simulink model "quad_nolinear"  (R2017b)
settings: Solver=VariableStepAuto  StartTime=0.0  StopTime=280  RelTol=1e-3
values from neighbouring files (symbols this model uses):
  A11 = Ab(1:6,1:6)    [quadrirrotor_ws.m]
  A12 = Ab(1:6,7:12)    [quadrirrotor_ws.m]
  A21 = Ab(7:12,1:6)    [quadrirrotor_ws.m]
  A22 = Ab(7:12,7:12)    [quadrirrotor_ws.m]
  Am = [zeros(6) eye(6); A_l zeros(6)]    [quadrirrotor_ws.m]
  B1 = Bb(1:6,:)    [quadrirrotor_ws.m]
  B2 = Bb(7:12,:)    [quadrirrotor_ws.m]
  Bm = [zeros(8,4); 1/m 0 0 0;0 1/Ixx 0 0;0 0 1/Iyy 0;0 0 0 1/Izz]    [quadrirrotor_ws.m]
  Cm = [eye(6) zeros(6)]    [quadrirrotor_ws.m]
  Dm = zeros(6,4)    [quadrirrotor_ws.m]
  g = 9.81    [quadrirrotor_ws.m]
  Ixx = 0.0363    [quadrirrotor_ws.m]
  Iyy = 0.0363    [quadrirrotor_ws.m]
  Izz = 0.0615    [quadrirrotor_ws.m]
  K = inv(R)*B'*P    [quadrirrotor_ws.m]
  Km = [zeros(6,12) ... (first row only)    [quadrirrotor_ws.m]
  Lb = inv(T)*Lc    [quadrirrotor_ws.m]
  m = 2.24    [quadrirrotor_ws.m]
  Y1 = Y(:,1:6)    [quadrirrotor_ws.m]
  Y2 = Y(:,7:12)    [quadrirrotor_ws.m]
libraries: simulink x4
settings Model: Creator=Italo  LastModifiedBy=Italo
settings OptimizationCC: LifeSpan=inf
settings DebuggingCC: SFExecutionAtInitializationDiag=none
settings CodeAppCC: StateflowObjectComments=on

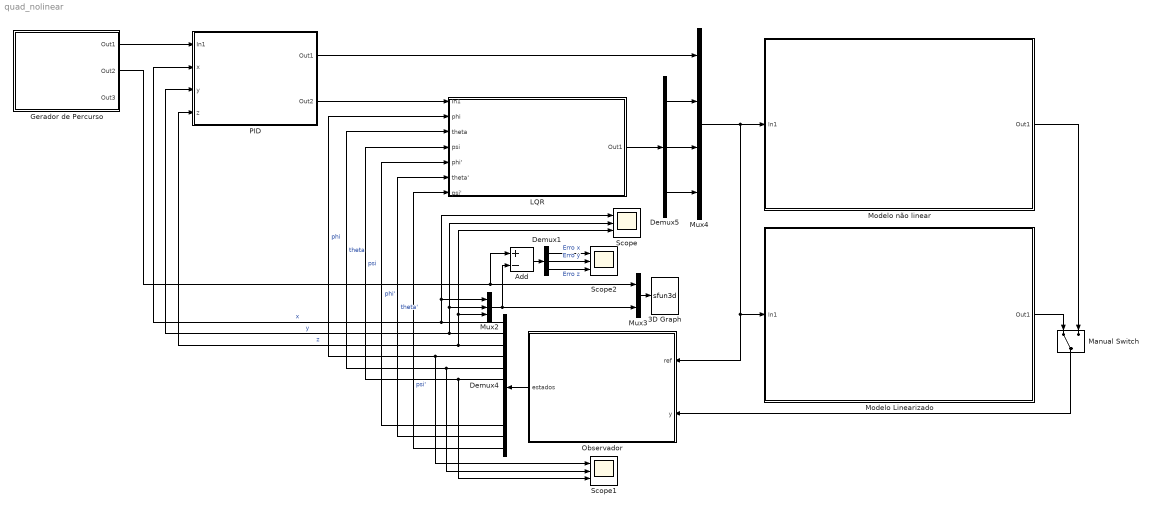
== system quad_nolinear ==
  3D Graph : S-Function  LoadFcn=if exist('sfun3d','file'), sfun3d([],[],[],'LoadBlock'); end  FunctionName=sfun3d  Parameters=ax,T,np,cp,gd,ls,mk,mx,hd,tb  SFunctionDeploymentMode=off  EnableBusSupport=off  mask(3D Graph){np=2, ax=[-5 5 -5 5 0 1500], mx=1e4, T=0.1, cp=[3 2 1], gd=on, hd=off, tb=off, ls=--, mk=none}
      mask prompts: np "Number of moving points (lines)"; ax "Range: [xmin xmax  ymin ymax zmin zmax]"; mx "Max number of points in each line"; T "Sampling Time"; cp "Camera position (use [0 0 1] for 2D XY view)"; gd "Grid (on|off)"; hd "HeadMarkers (on|off)"; tb "Toolbar (on|off)"; ls "LineStyle"; mk "LineMarker"
      mask help:
      | This block plots the position of several points in the XYZ space. The input contains the coordinates of all the points (x1,y1,z1,x2,y2,z2,...).
      | The number of moving points (lines), the XYZ ranges, sampling time, camera position, and grid (among other things) can be set as mask parameters.
      settings: CopyFcn=if exist('sfun3d','file'), sfun3d([],[],[],'CopyBlock'); end  DeleteFcn=if exist('sfun3d','file'), sfun3d([],[],[],'DeleteBlock'); end  NameChangeFcn=if exist('sfun3d','file'), sfun3d([],[],[],'NameChange'); end
      mask Help:
      | This block plots the position of several points in the XYZ space. The input contains the coordinates of all the points (x1,y1,z1,x2,y2,z2,...).
      | The number of moving points (lines), the XYZ ranges, sampling time, camera position, and grid (among other things) can be set as mask parameters.
      mask TypeOptions ls: - | -- | : | -. | none
      mask TypeOptions mk: none | . | + | o | * | x | square | diamond | v | ^ | > | < | pentagram | hexagram
      mask Display: plot([.05 .95 .95 .05 .05],[.45 .45 .95 .95 .45], 0.5+cos(0:0.1:2*pi)*0.3,0.7+sin(0:0.1:2*pi)*0.2)
  Add : Sum  Inputs=+-
  Demux1 : Demux  Outputs=3
  Demux4 : Demux  Outputs=12
  Demux5 : Demux  Outputs=3
  Gerador de Percurso : Subsystem
      mask Display: image('gerador.jpg');
  LQR : Subsystem
      mask Display: image('lqr.png');
  Manual Switch : ManualSwitch
  Modelo Linearizado : Subsystem
      mask Display: image('quadrotor.jpg');
  Modelo não linear : Subsystem
      mask Display: image('quadrotor.jpg');
  Mux2 : Mux  Inputs=3
  Mux3 : Mux  Inputs=2
  Mux4 : Mux
  Observador : Subsystem
      mask Display: image('observador.jpg');
  PID : Subsystem
      mask Display: image('pid.jpg');
  Scope : Scope  NumInputPorts=3
  Scope1 : Scope  NumInputPorts=3
  Scope2 : Scope  NumInputPorts=3
  wires:
  Demux5/3 -> Mux4/4
  Demux4/3 -> Mux2/3, Scope/3, PID/4(z)  "z"
  Demux4/6 -> Scope1/3, LQR/4(psi)  "psi"
  Demux4/2 -> Mux2/2, Scope/2, PID/3(y)  "y"
  Demux4/1 -> Mux2/1, Scope/1, PID/2(x)  "x"
  Demux5/1 -> Mux4/2
  Demux4/5 -> Scope1/2, LQR/3(theta)  "theta"
  Demux4/4 -> Scope1/1, LQR/2(phi)  "phi"
  Mux4/1 -> Observador/1(ref), Modelo Linearizado/1(In1), Modelo não linear/1(In1)
  Observador/1("estados ") -> Demux4/1
  Demux5/2 -> Mux4/3
  Manual Switch/1 -> Observador/2(y)
  Modelo Linearizado/1(Out1) -> Manual Switch/1
  Mux3/1 -> 3D Graph/1
  Mux2/1 -> Mux3/2, Add/2
  Gerador de Percurso/2(Out2) -> Add/1, Mux3/1
  Gerador de Percurso/1(Out1) -> PID/1(In1)
  PID/1(Out1) -> Mux4/1
  PID/2(Out2) -> LQR/1(In1)
  Demux4/10 -> LQR/5(phi')  "phi'"
  Demux4/11 -> LQR/6(theta')  "theta'"
  Demux4/12 -> LQR/7(psi')  "psi'"
  LQR/1(Out1) -> Demux5/1
  Add/1 -> Demux1/1
  Demux1/1 -> Scope2/1  "Erro x"
  Demux1/2 -> Scope2/2  "Erro y"
  Demux1/3 -> Scope2/3  "Erro z"
  Modelo não linear/1(Out1) -> Manual Switch/2

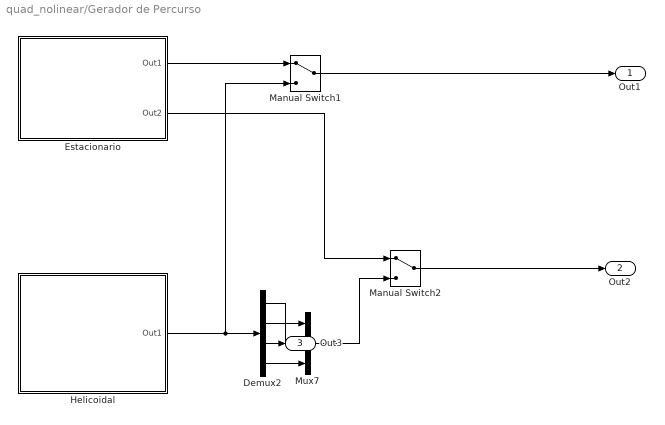
== system quad_nolinear/Gerador de Percurso ==
  Demux2 : Demux
  Estacionario : Subsystem
  Helicoidal : Subsystem
  Manual Switch1 : ManualSwitch
  Manual Switch2 : ManualSwitch
  Mux7 : Mux  Inputs=3
  Out1 : Outport
  Out2 : Outport  Port=2
  Out3 : Outport  Port=3
  wires:
  Manual Switch1/1 -> Out1/1
  Helicoidal/1(Out1) -> Manual Switch1/2, Demux2/1
  Manual Switch2/1 -> Out2/1
  Demux2/2 -> Mux7/1
  Demux2/3 -> Out3/1
  Demux2/4 -> Mux7/3
  Mux7/1 -> Manual Switch2/2
  Estacionario/1(Out1) -> Manual Switch1/1
  Estacionario/2(Out2) -> Manual Switch2/1
  Demux2/1 -> Mux7/2

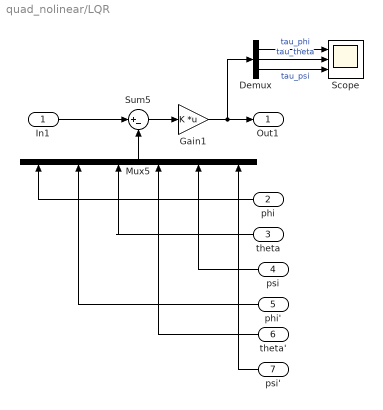
== system quad_nolinear/LQR ==
  In1 : Inport
  phi : Inport  Port=2
  theta : Inport  Port=3
  psi : Inport  Port=4
  phi' : Inport  Port=5
  theta' : Inport  Port=6
  psi' : Inport  Port=7
  Demux : Demux  Outputs=3
  Gain1 : Gain  Gain=K  Multiplication=Matrix(K*u) (u vector)
  Mux5 : Mux  Inputs=6
  Scope : Scope  NumInputPorts=3
  Sum5 : Sum  Inputs=|+-
  Out1 : Outport
  wires:
  theta/1 -> Mux5/3
  phi/1 -> Mux5/1
  psi/1 -> Mux5/5
  theta'/1 -> Mux5/4
  Sum5/1 -> Gain1/1
  psi'/1 -> Mux5/6
  phi'/1 -> Mux5/2
  Gain1/1 -> Demux/1, Out1/1
  Mux5/1 -> Sum5/2
  In1/1 -> Sum5/1
  Demux/1 -> Scope/1  "tau_phi"
  Demux/2 -> Scope/2  "tau_theta"
  Demux/3 -> Scope/3  "tau_psi"

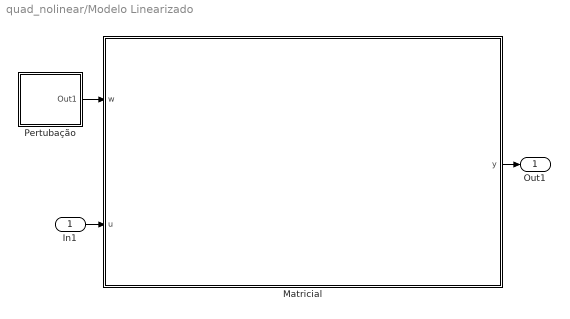
== system quad_nolinear/Modelo Linearizado ==
  In1 : Inport
  Matricial : Subsystem
  Pertubação : Subsystem
  Out1 : Outport
  wires:
  Pertubação/1(Out1) -> Matricial/1(w)
  In1/1 -> Matricial/2(u)
  Matricial/1(y) -> Out1/1

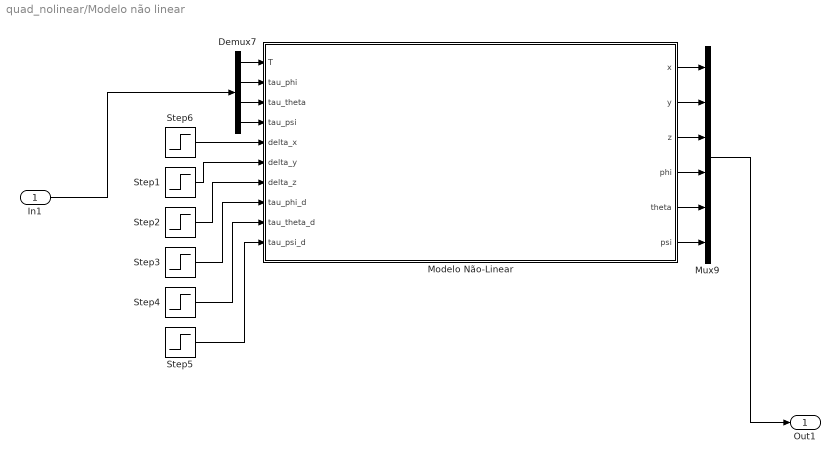
== system quad_nolinear/Modelo não linear ==
  In1 : Inport
  Demux7 : Demux
  Modelo Não-Linear : Subsystem
  Mux9 : Mux  Inputs=6
  Step1 : Step  Time=250  After=0.5  SampleTime=0
  Step2 : Step  Time=300  After=0.5  SampleTime=0
  Step3 : Step  Time=350  After=0.5  SampleTime=0
  Step4 : Step  Time=400  After=0.5  SampleTime=0
  Step5 : Step  Time=450  After=0.5  SampleTime=0
  Step6 : Step  Time=200  After=0.5  SampleTime=0
  Out1 : Outport
  wires:
  Modelo Não-Linear/1(x) -> Mux9/1
  In1/1 -> Demux7/1
  Step6/1 -> Modelo Não-Linear/5(delta_x)
  Step1/1 -> Modelo Não-Linear/6(delta_y)
  Step2/1 -> Modelo Não-Linear/7(delta_z)
  Step4/1 -> Modelo Não-Linear/9(tau_theta_d)
  Step5/1 -> Modelo Não-Linear/10(tau_psi_d)
  Step3/1 -> Modelo Não-Linear/8(tau_phi_d)
  Modelo Não-Linear/6(psi) -> Mux9/6
  Modelo Não-Linear/4(phi) -> Mux9/4
  Mux9/1 -> Out1/1
  Modelo Não-Linear/2(y) -> Mux9/2
  Modelo Não-Linear/3(z) -> Mux9/3
  Modelo Não-Linear/5(theta) -> Mux9/5
  Demux7/4 -> Modelo Não-Linear/4(tau_psi)
  Demux7/3 -> Modelo Não-Linear/3(tau_theta)
  Demux7/1 -> Modelo Não-Linear/1(T)
  Demux7/2 -> Modelo Não-Linear/2(tau_phi)

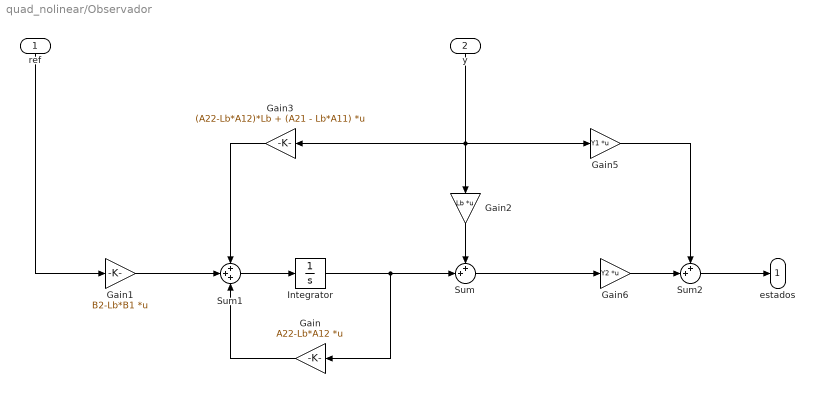
== system quad_nolinear/Observador ==
  ref : Inport
  y : Inport  Port=2
  Gain : Gain  Gain=A22-Lb*A12  Multiplication=Matrix(K*u) (u vector)
  Gain1 : Gain  Gain=B2-Lb*B1  Multiplication=Matrix(K*u) (u vector)
  Gain2 : Gain  Gain=Lb  Multiplication=Matrix(K*u) (u vector)
  Gain3 : Gain  Gain=(A22-Lb*A12)*Lb + (A21 - Lb*A11)  Multiplication=Matrix(K*u) (u vector)
  Gain5 : Gain  Gain=Y1  Multiplication=Matrix(K*u) (u vector)
  Gain6 : Gain  Gain=Y2  Multiplication=Matrix(K*u) (u vector)
  Integrator : Integrator
  Sum : Sum  Inputs=++|
  Sum1 : Sum  Inputs=+++
  Sum2 : Sum  Inputs=++|
  "estados " : Outport
  wires:
  Sum1/1 -> Integrator/1
  Integrator/1 -> Sum/2, Gain/1
  Gain/1 -> Sum1/3
  ref/1 -> Gain1/1
  Gain1/1 -> Sum1/2
  Gain3/1 -> Sum1/1
  y/1 -> Gain5/1, Gain3/1, Gain2/1
  Gain2/1 -> Sum/1
  Sum/1 -> Gain6/1
  Gain6/1 -> Sum2/2
  Sum2/1 -> "estados "/1
  Gain5/1 -> Sum2/1

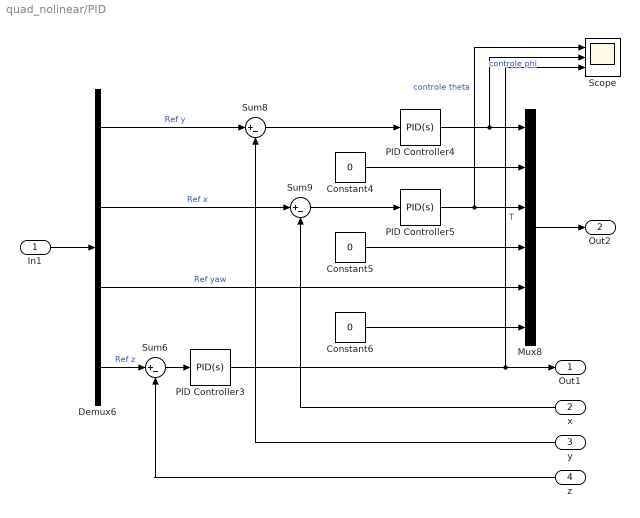
== system quad_nolinear/PID ==
  In1 : Inport
  x : Inport  Port=2
  y : Inport  Port=3
  z : Inport  Port=4
  Constant4 : Constant  Value=0
  Constant5 : Constant  Value=0
  Constant6 : Constant  Value=0
  Demux6 : Demux
  Mux8 : Mux  Inputs=6
  PID Controller3 : simulink/Continuous/PID Controller  Controller=PID  TimeDomain=Continuous-time  SampleTime=-1  IntegratorMethod=Forward Euler  FilterMethod=Forward Euler  Form=Ideal  UseFilter=on  ControllerParametersSource=internal  P=0.4  I=0.04  D=5.56  N=5.46  InitialConditionSource=internal  InitialConditionForIntegrator=0  InitialConditionForFilter=0  ExternalReset=none  LimitOutput=off  UpperSaturationLimit=inf  LowerSaturationLimit=-inf  LinearizeAsGain=on  AntiWindupMode=none  Kb=1  TrackingMode=off  Kt=1  PParamMin=[]  PParamMax=[]  IParamMin=[]  IParamMax=[]  DParamMin=[]  DParamMax=[]  NParamMin=[]  NParamMax=[]  KbParamMin=[]  KbParamMax=[]  KtParamMin=[]  KtParamMax=[]  POutMin=[]  POutMax=[]  IOutMin=[]  IOutMax=[]  DOutMin=[]  DOutMax=[]  NOutMin=[]  NOutMax=[]  KbOutMin=[]  KbOutMax=[]  KtOutMin=[]  KtOutMax=[]  IntegratorOutMin=[]  IntegratorOutMax=[]  FilterOutMin=[]  FilterOutMax=[]  SumOutMin=[]  SumOutMax=[]  SumI1OutMin=[]  SumI1OutMax=[]  SumI2OutMin=[]  SumI2OutMax=[]  SumI3OutMin=[]  SumI3OutMax=[]  SumDOutMin=[]  SumDOutMax=[]  SaturationOutMin=[]  SaturationOutMax=[]  IntegratorContinuousStateAttributes=''  IntegratorStateMustResolveToSignalObject=off  IntegratorRTWStateStorageClass=Auto  FilterContinuousStateAttributes=''  FilterStateMustResolveToSignalObject=off  FilterRTWStateStorageClass=Auto  DifferentiatorICPrevScaledInput=0  DifferentiatorOutMin=[]  DifferentiatorOutMax=[]  InitialConditionSetting=State (most efficient)  FilterDiffOutCoefMin=[]  FilterDiffOutCoefMax=[]  SumDenOutMin=[]  SumDenOutMax=[]  SumNumOutMin=[]  SumNumOutMax=[]  ReciprocalOutMin=[]  ReciprocalOutMax=[]  DivideOutMin=[]  DivideOutMax=[]  TunerSelectOption=Transfer Function Based (PID Tuner App)
  PID Controller4 : simulink/Continuous/PID Controller  Controller=PID  TimeDomain=Continuous-time  SampleTime=-1  IntegratorMethod=Forward Euler  FilterMethod=Forward Euler  Form=Ideal  UseFilter=on  ControllerParametersSource=internal  P=-0.01  I=0.01  D=30  N=140  InitialConditionSource=internal  InitialConditionForIntegrator=0  InitialConditionForFilter=0  ExternalReset=none  LimitOutput=off  UpperSaturationLimit=inf  LowerSaturationLimit=-inf  LinearizeAsGain=on  AntiWindupMode=none  Kb=1  TrackingMode=off  Kt=1  PParamMin=[]  PParamMax=[]  IParamMin=[]  IParamMax=[]  DParamMin=[]  DParamMax=[]  NParamMin=[]  NParamMax=[]  KbParamMin=[]  KbParamMax=[]  KtParamMin=[]  KtParamMax=[]  POutMin=[]  POutMax=[]  IOutMin=[]  IOutMax=[]  DOutMin=[]  DOutMax=[]  NOutMin=[]  NOutMax=[]  KbOutMin=[]  KbOutMax=[]  KtOutMin=[]  KtOutMax=[]  IntegratorOutMin=[]  IntegratorOutMax=[]  FilterOutMin=[]  FilterOutMax=[]  SumOutMin=[]  SumOutMax=[]  SumI1OutMin=[]  SumI1OutMax=[]  SumI2OutMin=[]  SumI2OutMax=[]  SumI3OutMin=[]  SumI3OutMax=[]  SumDOutMin=[]  SumDOutMax=[]  SaturationOutMin=[]  SaturationOutMax=[]  IntegratorContinuousStateAttributes=''  IntegratorStateMustResolveToSignalObject=off  IntegratorRTWStateStorageClass=Auto  FilterContinuousStateAttributes=''  FilterStateMustResolveToSignalObject=off  FilterRTWStateStorageClass=Auto  DifferentiatorICPrevScaledInput=0  DifferentiatorOutMin=[]  DifferentiatorOutMax=[]  InitialConditionSetting=State (most efficient)  FilterDiffOutCoefMin=[]  FilterDiffOutCoefMax=[]  SumDenOutMin=[]  SumDenOutMax=[]  SumNumOutMin=[]  SumNumOutMax=[]  ReciprocalOutMin=[]  ReciprocalOutMax=[]  DivideOutMin=[]  DivideOutMax=[]  TunerSelectOption=Transfer Function Based (PID Tuner App)
  PID Controller5 : simulink/Continuous/PID Controller  Controller=PID  TimeDomain=Continuous-time  SampleTime=-1  IntegratorMethod=Forward Euler  FilterMethod=Forward Euler  Form=Ideal  UseFilter=on  ControllerParametersSource=internal  P=0.001  I=0.003  D=60  N=58  InitialConditionSource=internal  InitialConditionForIntegrator=0  InitialConditionForFilter=0  ExternalReset=none  LimitOutput=off  UpperSaturationLimit=inf  LowerSaturationLimit=-inf  LinearizeAsGain=on  AntiWindupMode=none  Kb=1  TrackingMode=off  Kt=1  PParamMin=[]  PParamMax=[]  IParamMin=[]  IParamMax=[]  DParamMin=[]  DParamMax=[]  NParamMin=[]  NParamMax=[]  KbParamMin=[]  KbParamMax=[]  KtParamMin=[]  KtParamMax=[]  POutMin=[]  POutMax=[]  IOutMin=[]  IOutMax=[]  DOutMin=[]  DOutMax=[]  NOutMin=[]  NOutMax=[]  KbOutMin=[]  KbOutMax=[]  KtOutMin=[]  KtOutMax=[]  IntegratorOutMin=[]  IntegratorOutMax=[]  FilterOutMin=[]  FilterOutMax=[]  SumOutMin=[]  SumOutMax=[]  SumI1OutMin=[]  SumI1OutMax=[]  SumI2OutMin=[]  SumI2OutMax=[]  SumI3OutMin=[]  SumI3OutMax=[]  SumDOutMin=[]  SumDOutMax=[]  SaturationOutMin=[]  SaturationOutMax=[]  IntegratorContinuousStateAttributes=''  IntegratorStateMustResolveToSignalObject=off  IntegratorRTWStateStorageClass=Auto  FilterContinuousStateAttributes=''  FilterStateMustResolveToSignalObject=off  FilterRTWStateStorageClass=Auto  DifferentiatorICPrevScaledInput=0  DifferentiatorOutMin=[]  DifferentiatorOutMax=[]  InitialConditionSetting=State (most efficient)  FilterDiffOutCoefMin=[]  FilterDiffOutCoefMax=[]  SumDenOutMin=[]  SumDenOutMax=[]  SumNumOutMin=[]  SumNumOutMax=[]  ReciprocalOutMin=[]  ReciprocalOutMax=[]  DivideOutMin=[]  DivideOutMax=[]  TunerSelectOption=Transfer Function Based (PID Tuner App)
  Scope : Scope  NumInputPorts=3
  Sum6 : Sum  Inputs=|+-
  Sum8 : Sum  Inputs=|+-
  Sum9 : Sum  Inputs=|+-
  Out1 : Outport
  Out2 : Outport  Port=2
  wires:
  Demux6/2 -> Sum9/1  "Ref x"
  Demux6/4 -> Sum6/1  "Ref z"
  Mux8/1 -> Out2/1
  Sum9/1 -> PID Controller5/1
  Constant4/1 -> Mux8/2
  Demux6/1 -> Sum8/1  "Ref y"
  PID Controller3/1 -> Scope/3, Out1/1  "T"
  Sum6/1 -> PID Controller3/1
  Constant6/1 -> Mux8/6
  Constant5/1 -> Mux8/4
  Demux6/3 -> Mux8/5  "Ref yaw"
  Sum8/1 -> PID Controller4/1
  In1/1 -> Demux6/1
  PID Controller4/1 -> Scope/2, Mux8/1  "controle phi"
  y/1 -> Sum8/2
  x/1 -> Sum9/2
  z/1 -> Sum6/2
  PID Controller5/1 -> Scope/1, Mux8/3  "controle theta"

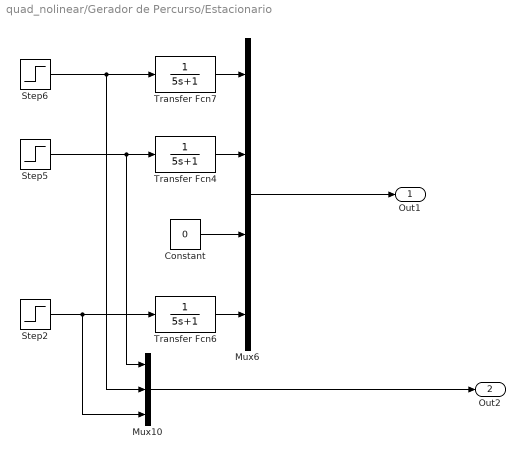
== system quad_nolinear/Gerador de Percurso/Estacionario ==
  Constant : Constant  Value=0
  Mux10 : Mux  Inputs=3
  Mux6 : Mux
  Step2 : Step  After=10  SampleTime=0
  Step5 : Step  After=2  SampleTime=0
  Step6 : Step  After=2  SampleTime=0
  Transfer Fcn4 : TransferFcn  Denominator=[5 1]
  Transfer Fcn6 : TransferFcn  Denominator=[5 1]
  Transfer Fcn7 : TransferFcn  Denominator=[5 1]
  Out1 : Outport
  Out2 : Outport  Port=2
  wires:
  Mux10/1 -> Out2/1
  Step2/1 -> Mux10/3, Transfer Fcn6/1
  Constant/1 -> Mux6/3
  Transfer Fcn7/1 -> Mux6/1
  Transfer Fcn4/1 -> Mux6/2
  Step6/1 -> Mux10/2, Transfer Fcn7/1
  Transfer Fcn6/1 -> Mux6/4
  Step5/1 -> Mux10/1, Transfer Fcn4/1
  Mux6/1 -> Out1/1

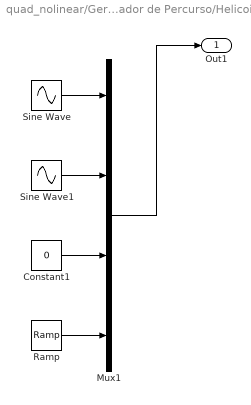
== system quad_nolinear/Gerador de Percurso/Helicoidal ==
  Constant1 : Constant  Value=0
  Mux1 : Mux
  Ramp : simulink/Sources/Ramp  slope=3  start=0  X0=1
  Sine Wave : Sin  Amplitude=3  Frequency=0.1  SampleTime=0
  Sine Wave1 : Sin  Amplitude=3  Frequency=0.1  Phase=pi/2  SampleTime=0
  Out1 : Outport
  wires:
  Sine Wave1/1 -> Mux1/2
  Sine Wave/1 -> Mux1/1
  Ramp/1 -> Mux1/4
  Mux1/1 -> Out1/1
  Constant1/1 -> Mux1/3

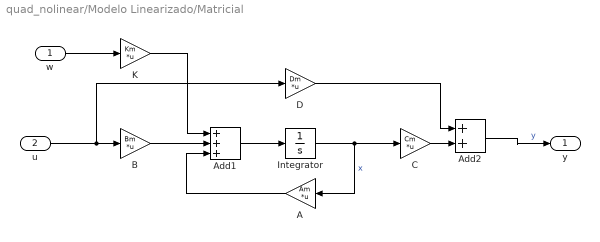
== system quad_nolinear/Modelo Linearizado/Matricial ==
  w : Inport
  u : Inport  Port=2
  A : Gain  Gain=Am  Multiplication=Matrix(K*u) (u vector)
  Add1 : Sum  Inputs=+++
  Add2 : Sum
  B : Gain  Gain=Bm  Multiplication=Matrix(K*u) (u vector)
  C : Gain  Gain=Cm  Multiplication=Matrix(K*u) (u vector)
  D : Gain  Gain=Dm  Multiplication=Matrix(K*u) (u vector)
  Integrator : Integrator
  K : Gain  Gain=Km  Multiplication=Matrix(K*u) (u vector)
  y : Outport
  wires:
  u/1 -> D/1, B/1
  Add2/1 -> y/1  "y"
  B/1 -> Add1/2
  Integrator/1 -> A/1, C/1  "x"
  A/1 -> Add1/3
  K/1 -> Add1/1
  D/1 -> Add2/1
  w/1 -> K/1
  Add1/1 -> Integrator/1
  C/1 -> Add2/2

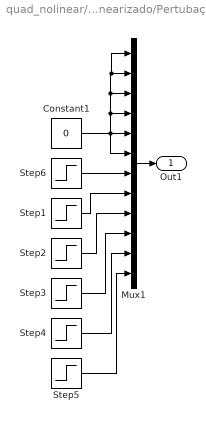
== system quad_nolinear/Modelo Linearizado/Pertubação ==
  Constant1 : Constant  Value=0
  Mux1 : Mux  Inputs=12
  Step1 : Step  Time=250  After=0.01  SampleTime=0
  Step2 : Step  Time=300  After=0.01  SampleTime=0
  Step3 : Step  Time=350  After=0.01  SampleTime=0
  Step4 : Step  Time=400  After=0.01  SampleTime=0
  Step5 : Step  Time=450  After=0.01  SampleTime=0
  Step6 : Step  Time=200  After=0.01  SampleTime=0
  Out1 : Outport
  wires:
  Step2/1 -> Mux1/9
  Step5/1 -> Mux1/12
  Mux1/1 -> Out1/1
  Constant1/1 -> Mux1/6, Mux1/1, Mux1/2, Mux1/3, Mux1/4, Mux1/5
  Step3/1 -> Mux1/10
  Step6/1 -> Mux1/7
  Step4/1 -> Mux1/11
  Step1/1 -> Mux1/8

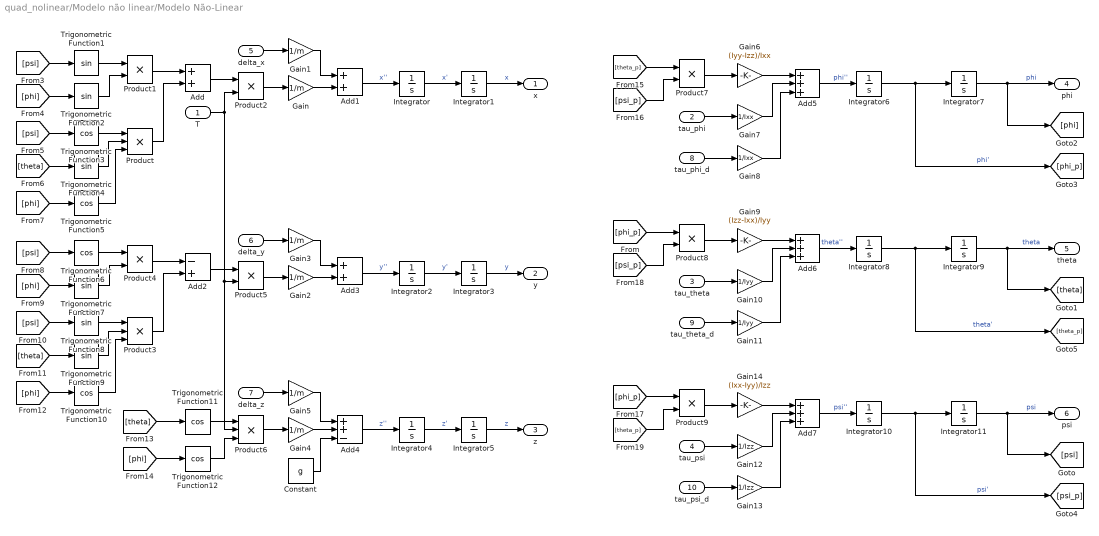
== system quad_nolinear/Modelo não linear/Modelo Não-Linear ==
  T : Inport
  tau_phi : Inport  Port=2
  tau_theta : Inport  Port=3
  tau_psi : Inport  Port=4
  delta_x : Inport  Port=5
  delta_y : Inport  Port=6
  delta_z : Inport  Port=7
  tau_phi_d : Inport  Port=8
  tau_theta_d : Inport  Port=9
  tau_psi_d : Inport  Port=10
  Add : Sum
  Add1 : Sum
  Add2 : Sum  Inputs=-+
  Add3 : Sum
  Add4 : Sum  Inputs=++-
  Add5 : Sum  Inputs=+++
  Add6 : Sum  Inputs=+++
  Add7 : Sum  Inputs=+++
  Constant : Constant  Value=g
  Gain{,1..5} (6 alike) : Gain  Gain=1/m
  Gain10 : Gain  Gain=1/Iyy
  Gain11 : Gain  Gain=1/Iyy
  Gain12 : Gain  Gain=1/Izz
  Gain13 : Gain  Gain=1/Izz
  Gain14 : Gain  Gain=(Ixx-Iyy)/Izz
  Gain6 : Gain  Gain=(Iyy-Izz)/Ixx
  Gain7 : Gain  Gain=1/Ixx
  Gain8 : Gain  Gain=1/Ixx
  Gain9 : Gain  Gain=(Izz-Ixx)/Iyy
  Integrator{,1..11} (12 alike) : Integrator
  Product : Product  Inputs=3
  Product{1..2,4..5,7..9} (7 alike) : Product
  Product3 : Product  Inputs=3
  Product6 : Product  Inputs=3
  Trigonometric Function{1..2,4,7..9} (6 alike) : Trigonometry
  Trigonometric Function{3,5..6,10..12} (6 alike) : Trigonometry  Operator=cos
  x : Outport
  y : Outport  Port=2
  z : Outport  Port=3
  phi : Outport  Port=4
  theta : Outport  Port=5
  psi : Outport  Port=6
  wires:
  Integrator/1 -> Integrator1/1  "x'"
  Integrator1/1 -> x/1  "x"
  Trigonometric Function1/1 -> Product1/1
  Trigonometric Function2/1 -> Product1/2
  [psi] -> Trigonometric Function1/1
  [phi] -> Trigonometric Function2/1
  Trigonometric Function3/1 -> Product/1
  [psi] -> Trigonometric Function3/1
  Trigonometric Function4/1 -> Product/2
  [theta] -> Trigonometric Function4/1
  Trigonometric Function5/1 -> Product/3
  [phi] -> Trigonometric Function5/1
  Product1/1 -> Add/1
  Product/1 -> Add/2
  Add/1 -> Product2/1
  Product2/1 -> Gain/1
  Gain/1 -> Add1/2
  Gain1/1 -> Add1/1
  Add1/1 -> Integrator/1  "x''"
  Integrator2/1 -> Integrator3/1  "y'"
  [psi] -> Trigonometric Function8/1
  Trigonometric Function9/1 -> Product3/2
  Product4/1 -> Add2/1
  [theta] -> Trigonometric Function9/1
  Add3/1 -> Integrator2/1  "y''"
  Trigonometric Function6/1 -> Product4/1
  Trigonometric Function10/1 -> Product3/3
  [psi] -> Trigonometric Function6/1
  Trigonometric Function7/1 -> Product4/2
  Gain2/1 -> Add3/2
  Product5/1 -> Gain2/1
  Integrator3/1 -> y/1  "y"
  [phi] -> Trigonometric Function10/1
  Product3/1 -> Add2/2
  Gain3/1 -> Add3/1
  Add2/1 -> Product5/1
  [phi] -> Trigonometric Function7/1
  Trigonometric Function8/1 -> Product3/1
  Product6/1 -> Gain4/1
  Add4/1 -> Integrator4/1  "z''"
  Gain4/1 -> Add4/2
  T/1 -> Product6/2, Product5/2, Product2/2
  Gain5/1 -> Add4/1
  Integrator4/1 -> Integrator5/1  "z'"
  Trigonometric Function11/1 -> Product6/1
  Integrator5/1 -> z/1  "z"
  Constant/1 -> Add4/3
  Trigonometric Function12/1 -> Product6/3
  [theta] -> Trigonometric Function11/1
  [phi] -> Trigonometric Function12/1
  Add5/1 -> Integrator6/1  "phi''"
  Integrator7/1 -> [phi], phi/1  "phi"
  Integrator6/1 -> Integrator7/1, [phi_p]  "phi'"
  Product7/1 -> Gain6/1
  Gain6/1 -> Add5/1
  [theta_p] -> Product7/1
  [psi_p] -> Product7/2
  Gain7/1 -> Add5/2
  tau_phi/1 -> Gain7/1
  Gain8/1 -> Add5/3
  Integrator8/1 -> [theta_p], Integrator9/1  "theta'"
  Integrator9/1 -> [theta], theta/1  "theta"
  [phi_p] -> Product8/1
  tau_theta/1 -> Gain10/1
  Add6/1 -> Integrator8/1  "theta''"
  Product8/1 -> Gain9/1
  Gain10/1 -> Add6/2
  Gain9/1 -> Add6/1
  [psi_p] -> Product8/2
  Gain11/1 -> Add6/3
  Gain13/1 -> Add7/3
  Product9/1 -> Gain14/1
  [theta_p] -> Product9/2
  Gain12/1 -> Add7/2
  Add7/1 -> Integrator10/1  "psi''"
  Integrator11/1 -> [psi], psi/1  "psi"
  Integrator10/1 -> [psi_p], Integrator11/1  "psi'"
  Gain14/1 -> Add7/1
  tau_psi/1 -> Gain12/1
  [phi_p] -> Product9/1
  delta_x/1 -> Gain1/1
  delta_y/1 -> Gain3/1
  delta_z/1 -> Gain5/1
  tau_phi_d/1 -> Gain8/1
  tau_theta_d/1 -> Gain11/1
  tau_psi_d/1 -> Gain13/1
